simulink model "ClosedLoop_ACCsim"  (Simulink 9.2)
settings: Solver=VariableStepAuto  StartTime=0.0  StopTime=5  RelTol=1e-3
libraries: neural x533
(part 10 of 24)

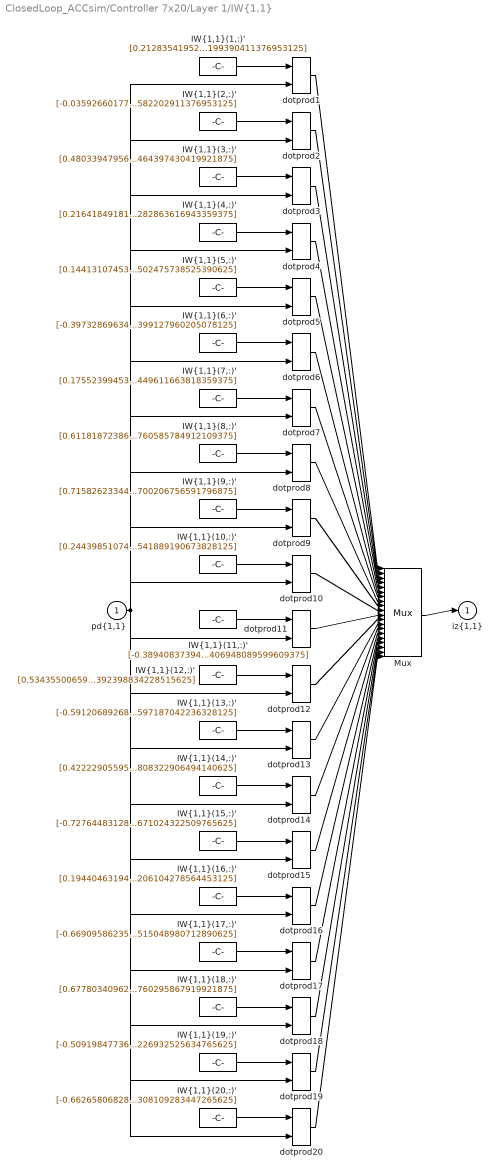
== system ClosedLoop_ACCsim/Controller 7x20/Layer 1/IW{1,1} ==
  "pd{1,1}" : Inport  PortDimensions=5
      mask Display: e = 0.06;c1 = [120 230 180]/255;c2 = ([120 230 180]+0)/(256+128);c3 = ([120 230 180]+128)/(256+128);patch([0 1 1 0],[0 0 1 1],c1);patch([0 1 1 1-e 1-e 0+e],[0 0 1 1-e 0+e 0+e],c2);patch([0 0 1 1-e 0+e 0+e],[0 1 1 1-e 1-e 0+e],c3);plot([0 1 1 0 0],[0 0 1 1 0]);
  "IW{1,1}(1,:)'" : Constant  Value=[0.212835419521011315335812241755775175988674163818359375;-0.3927359580132747662872816363233141601085662841796875;-0.144152301067769827991327247218578122556209564208984375;-0.58889119361664221674601549239014275372028350830078125;-0.034369251210462976875437135504398611374199390411376953125]
      mask Display: e = 0.06;c1 = [120 150 230]/255;c2 = ([120 150 230]+0)/383;c3 = ([120 150 230]+128)/383;patch([0 1 1 0],[0 0 1 1],c1);patch([0 1 1 1-e 1-e 0+e],[0 0 1 1-e 0+e 0+e],c2);patch([0 0 1 1-e 0+e 0+e],[0 1 1 1-e 1-e 0+e],c3);plot([0 1 1 0 0],[0 0 1 1 0]);disp('Weights');
  "IW{1,1}(10,:)'" : Constant  Value=[0.2443985107421249580728073169666458852589130401611328125;0.251248156472832884222867733114981092512607574462890625;0.12802800348474974168055950940470211207866668701171875;0.5142082099368210368339759952505119144916534423828125;0.295116604969453633078302345893462188541889190673828125]
      mask Display: e = 0.06;c1 = [120 150 230]/255;c2 = ([120 150 230]+0)/383;c3 = ([120 150 230]+128)/383;patch([0 1 1 0],[0 0 1 1],c1);patch([0 1 1 1-e 1-e 0+e],[0 0 1 1-e 0+e 0+e],c2);patch([0 0 1 1-e 0+e 0+e],[0 1 1 1-e 1-e 0+e],c3);plot([0 1 1 0 0],[0 0 1 1 0]);disp('Weights');
  "IW{1,1}(11,:)'" : Constant  Value=[-0.389408373941988517064061170458444394171237945556640625;-0.5598485732379170354278130616876296699047088623046875;0.18512337722791460947746600140817463397979736328125;0.15592881193242147386257556718192063271999359130859375;-0.56991107693016029855925808078609406948089599609375]
      mask Display: e = 0.06;c1 = [120 150 230]/255;c2 = ([120 150 230]+0)/383;c3 = ([120 150 230]+128)/383;patch([0 1 1 0],[0 0 1 1],c1);patch([0 1 1 1-e 1-e 0+e],[0 0 1 1-e 0+e 0+e],c2);patch([0 0 1 1-e 0+e 0+e],[0 1 1 1-e 1-e 0+e],c3);plot([0 1 1 0 0],[0 0 1 1 0]);disp('Weights');
  "IW{1,1}(12,:)'" : Constant  Value=[0.5343550065999895792856477783061563968658447265625;0.250744758001088363652542057025129906833171844482421875;-0.461235807435400213538656544187688268721103668212890625;0.1640473631794022446594993880353285931050777435302734375;0.67067318966512046163330751369358040392398834228515625]
      mask Display: e = 0.06;c1 = [120 150 230]/255;c2 = ([120 150 230]+0)/383;c3 = ([120 150 230]+128)/383;patch([0 1 1 0],[0 0 1 1],c1);patch([0 1 1 1-e 1-e 0+e],[0 0 1 1-e 0+e 0+e],c2);patch([0 0 1 1-e 0+e 0+e],[0 1 1 1-e 1-e 0+e],c3);plot([0 1 1 0 0],[0 0 1 1 0]);disp('Weights');
  "IW{1,1}(13,:)'" : Constant  Value=[-0.5912068926854825434702433994971215724945068359375;-0.2038470656672795866537484243963262997567653656005859375;-0.1583124425194095408198080576767097227275371551513671875;-0.486613579148853225841975245202775113284587860107421875;-0.1335803269614399824138928352112998254597187042236328125]
      mask Display: e = 0.06;c1 = [120 150 230]/255;c2 = ([120 150 230]+0)/383;c3 = ([120 150 230]+128)/383;patch([0 1 1 0],[0 0 1 1],c1);patch([0 1 1 1-e 1-e 0+e],[0 0 1 1-e 0+e 0+e],c2);patch([0 0 1 1-e 0+e 0+e],[0 1 1 1-e 1-e 0+e],c3);plot([0 1 1 0 0],[0 0 1 1 0]);disp('Weights');
  "IW{1,1}(14,:)'" : Constant  Value=[0.4222290559586252545187790019554086029529571533203125;0.589193425221622657517173138330690562725067138671875;0.5154792487456205662965658120810985565185546875;-0.44820131779535354876742303531500510871410369873046875;-0.028408822728697803727815340835149982012808322906494140625]
      mask Display: e = 0.06;c1 = [120 150 230]/255;c2 = ([120 150 230]+0)/383;c3 = ([120 150 230]+128)/383;patch([0 1 1 0],[0 0 1 1],c1);patch([0 1 1 1-e 1-e 0+e],[0 0 1 1-e 0+e 0+e],c2);patch([0 0 1 1-e 0+e 0+e],[0 1 1 1-e 1-e 0+e],c3);plot([0 1 1 0 0],[0 0 1 1 0]);disp('Weights');
  "IW{1,1}(15,:)'" : Constant  Value=[-0.72764483128828494340467614165390841662883758544921875;0.76631521718359596473391093240934424102306365966796875;-0.261586670059799575316361597288050688803195953369140625;0.26312492002977949656639111708500422537326812744140625;0.90935896357760359620669987634755671024322509765625]
      mask Display: e = 0.06;c1 = [120 150 230]/255;c2 = ([120 150 230]+0)/383;c3 = ([120 150 230]+128)/383;patch([0 1 1 0],[0 0 1 1],c1);patch([0 1 1 1-e 1-e 0+e],[0 0 1 1-e 0+e 0+e],c2);patch([0 0 1 1-e 0+e 0+e],[0 1 1 1-e 1-e 0+e],c3);plot([0 1 1 0 0],[0 0 1 1 0]);disp('Weights');
  "IW{1,1}(16,:)'" : Constant  Value=[0.194404631947168893280064594364375807344913482666015625;0.5552546495174126572891282194177620112895965576171875;0.058508554392630300611255478315797518007457256317138671875;-0.27216863837114579904863376214052550494670867919921875;0.7418254711021508018831127628800459206104278564453125]
      mask Display: e = 0.06;c1 = [120 150 230]/255;c2 = ([120 150 230]+0)/383;c3 = ([120 150 230]+128)/383;patch([0 1 1 0],[0 0 1 1],c1);patch([0 1 1 1-e 1-e 0+e],[0 0 1 1-e 0+e 0+e],c2);patch([0 0 1 1-e 0+e 0+e],[0 1 1 1-e 1-e 0+e],c3);plot([0 1 1 0 0],[0 0 1 1 0]);disp('Weights');
  "IW{1,1}(17,:)'" : Constant  Value=[-0.6690958623540581573507779467036016285419464111328125;0.414850507163107007357893962762318551540374755859375;0.36526786443267000858980964039801619946956634521484375;0.066989067247426092865936197995324619114398956298828125;0.492191258252048735588601857671164907515048980712890625]
      mask Display: e = 0.06;c1 = [120 150 230]/255;c2 = ([120 150 230]+0)/383;c3 = ([120 150 230]+128)/383;patch([0 1 1 0],[0 0 1 1],c1);patch([0 1 1 1-e 1-e 0+e],[0 0 1 1-e 0+e 0+e],c2);patch([0 0 1 1-e 0+e 0+e],[0 1 1 1-e 1-e 0+e],c3);plot([0 1 1 0 0],[0 0 1 1 0]);disp('Weights');
  "IW{1,1}(18,:)'" : Constant  Value=[0.67780340962930984982648396908189170062541961669921875;-0.166200801785160667822793811865267343819141387939453125;0.007773451654268163750483022766957219573669135570526123046875;-0.6277118496053983864868541786563582718372344970703125;-0.10179050764502566017721818525387789122760295867919921875]
      mask Display: e = 0.06;c1 = [120 150 230]/255;c2 = ([120 150 230]+0)/383;c3 = ([120 150 230]+128)/383;patch([0 1 1 0],[0 0 1 1],c1);patch([0 1 1 1-e 1-e 0+e],[0 0 1 1-e 0+e 0+e],c2);patch([0 0 1 1-e 0+e 0+e],[0 1 1 1-e 1-e 0+e],c3);plot([0 1 1 0 0],[0 0 1 1 0]);disp('Weights');
  "IW{1,1}(19,:)'" : Constant  Value=[-0.50919847736597778631306709939963184297084808349609375;0.29458849558637767440671950680552981793880462646484375;0.6164242054481239296848116282490082085132598876953125;-0.05022444481905320723402752491892897523939609527587890625;0.56929857309828568734388909433619119226932525634765625]
      mask Display: e = 0.06;c1 = [120 150 230]/255;c2 = ([120 150 230]+0)/383;c3 = ([120 150 230]+128)/383;patch([0 1 1 0],[0 0 1 1],c1);patch([0 1 1 1-e 1-e 0+e],[0 0 1 1-e 0+e 0+e],c2);patch([0 0 1 1-e 0+e 0+e],[0 1 1 1-e 1-e 0+e],c3);plot([0 1 1 0 0],[0 0 1 1 0]);disp('Weights');
  "IW{1,1}(2,:)'" : Constant  Value=[-0.035926601776865262072302442675209022127091884613037109375;0.341274893573676296743002467337646521627902984619140625;-0.1624957466411529605210262161563150584697723388671875;0.68546422590090638760074170932057313621044158935546875;-0.76852906292452705105944232855108566582202911376953125]
      mask Display: e = 0.06;c1 = [120 150 230]/255;c2 = ([120 150 230]+0)/383;c3 = ([120 150 230]+128)/383;patch([0 1 1 0],[0 0 1 1],c1);patch([0 1 1 1-e 1-e 0+e],[0 0 1 1-e 0+e 0+e],c2);patch([0 0 1 1-e 0+e 0+e],[0 1 1 1-e 1-e 0+e],c3);plot([0 1 1 0 0],[0 0 1 1 0]);disp('Weights');
  "IW{1,1}(20,:)'" : Constant  Value=[-0.66265806828597562105898077788879163563251495361328125;-0.8358574702130796563182002500980161130428314208984375;0.332826348998758014818832862147246487438678741455078125;0.75074131206823901951707966873073019087314605712890625;-0.1851004659156537945907672337853000499308109283447265625]
      mask Display: e = 0.06;c1 = [120 150 230]/255;c2 = ([120 150 230]+0)/383;c3 = ([120 150 230]+128)/383;patch([0 1 1 0],[0 0 1 1],c1);patch([0 1 1 1-e 1-e 0+e],[0 0 1 1-e 0+e 0+e],c2);patch([0 0 1 1-e 0+e 0+e],[0 1 1 1-e 1-e 0+e],c3);plot([0 1 1 0 0],[0 0 1 1 0]);disp('Weights');
  "IW{1,1}(3,:)'" : Constant  Value=[0.480339479563791471594669246769626624882221221923828125;-0.59592850278037456934754345638793893158435821533203125;-0.1930903352979157772129070735900313593447208404541015625;0.114496074419272619859810902198660187423229217529296875;-0.361143691370916009031333260281826369464397430419921875]
      mask Display: e = 0.06;c1 = [120 150 230]/255;c2 = ([120 150 230]+0)/383;c3 = ([120 150 230]+128)/383;patch([0 1 1 0],[0 0 1 1],c1);patch([0 1 1 1-e 1-e 0+e],[0 0 1 1-e 0+e 0+e],c2);patch([0 0 1 1-e 0+e 0+e],[0 1 1 1-e 1-e 0+e],c3);plot([0 1 1 0 0],[0 0 1 1 0]);disp('Weights');
  "IW{1,1}(4,:)'" : Constant  Value=[0.2164184918114815114886795299753430299460887908935546875;0.9400873566467999875584382607485167682170867919921875;-0.303205328969188225851638662788900546729564666748046875;-0.44570874540381921757870031797210685908794403076171875;0.18120949337870850825993329635821282863616943359375]
      mask Display: e = 0.06;c1 = [120 150 230]/255;c2 = ([120 150 230]+0)/383;c3 = ([120 150 230]+128)/383;patch([0 1 1 0],[0 0 1 1],c1);patch([0 1 1 1-e 1-e 0+e],[0 0 1 1-e 0+e 0+e],c2);patch([0 0 1 1-e 0+e 0+e],[0 1 1 1-e 1-e 0+e],c3);plot([0 1 1 0 0],[0 0 1 1 0]);disp('Weights');
  "IW{1,1}(5,:)'" : Constant  Value=[0.1441310745332750331559878986809053458273410797119140625;-0.9206317506257928329205242334865033626556396484375;-0.4099304221757520405589048095862381160259246826171875;-0.568009386779689151580896577797830104827880859375;0.344113066470443096367404223201447166502475738525390625]
      mask Display: e = 0.06;c1 = [120 150 230]/255;c2 = ([120 150 230]+0)/383;c3 = ([120 150 230]+128)/383;patch([0 1 1 0],[0 0 1 1],c1);patch([0 1 1 1-e 1-e 0+e],[0 0 1 1-e 0+e 0+e],c2);patch([0 0 1 1-e 0+e 0+e],[0 1 1 1-e 1-e 0+e],c3);plot([0 1 1 0 0],[0 0 1 1 0]);disp('Weights');
  "IW{1,1}(6,:)'" : Constant  Value=[-0.397328696346857801469099058522260747849941253662109375;-0.0029566435601016071398061679786906097433529794216156005859375;0.4309051632885638749570489380857907235622406005859375;-0.67053491722794689167130854912102222442626953125;-0.466971235009332463761211329256184399127960205078125]
      mask Display: e = 0.06;c1 = [120 150 230]/255;c2 = ([120 150 230]+0)/383;c3 = ([120 150 230]+128)/383;patch([0 1 1 0],[0 0 1 1],c1);patch([0 1 1 1-e 1-e 0+e],[0 0 1 1-e 0+e 0+e],c2);patch([0 0 1 1-e 0+e 0+e],[0 1 1 1-e 1-e 0+e],c3);plot([0 1 1 0 0],[0 0 1 1 0]);disp('Weights');
  "IW{1,1}(7,:)'" : Constant  Value=[0.175523994536887883999298765047569759190082550048828125;0.2783338599097124888004373133298940956592559814453125;0.67569683197213648018220055746496655046939849853515625;-0.84534829514369536074269717573770321905612945556640625;0.08340677879841050523790357829057029448449611663818359375]
      mask Display: e = 0.06;c1 = [120 150 230]/255;c2 = ([120 150 230]+0)/383;c3 = ([120 150 230]+128)/383;patch([0 1 1 0],[0 0 1 1],c1);patch([0 1 1 1-e 1-e 0+e],[0 0 1 1-e 0+e 0+e],c2);patch([0 0 1 1-e 0+e 0+e],[0 1 1 1-e 1-e 0+e],c3);plot([0 1 1 0 0],[0 0 1 1 0]);disp('Weights');
  "IW{1,1}(8,:)'" : Constant  Value=[0.61181872386841373856469772363197989761829376220703125;-0.201160270514594896607007967759273014962673187255859375;0.377397473828878116108853646437637507915496826171875;-0.22875332743301834970139907454722560942173004150390625;0.1859440325483736611289486972964368760585784912109375]
      mask Display: e = 0.06;c1 = [120 150 230]/255;c2 = ([120 150 230]+0)/383;c3 = ([120 150 230]+128)/383;patch([0 1 1 0],[0 0 1 1],c1);patch([0 1 1 1-e 1-e 0+e],[0 0 1 1-e 0+e 0+e],c2);patch([0 0 1 1-e 0+e 0+e],[0 1 1 1-e 1-e 0+e],c3);plot([0 1 1 0 0],[0 0 1 1 0]);disp('Weights');
  "IW{1,1}(9,:)'" : Constant  Value=[0.71582623344398610409911043461761437356472015380859375;-0.897528066616040565151024566148407757282257080078125;-0.715669583388752972297197629814036190509796142578125;0.052208333596294072276311482028177124448120594024658203125;0.254905335750240158443347127104061655700206756591796875]
      mask Display: e = 0.06;c1 = [120 150 230]/255;c2 = ([120 150 230]+0)/383;c3 = ([120 150 230]+128)/383;patch([0 1 1 0],[0 0 1 1],c1);patch([0 1 1 1-e 1-e 0+e],[0 0 1 1-e 0+e 0+e],c2);patch([0 0 1 1-e 0+e 0+e],[0 1 1 1-e 1-e 0+e],c3);plot([0 1 1 0 0],[0 0 1 1 0]);disp('Weights');
  Mux : Mux  Inputs=20
      mask Display: e = 0.06;c1 = [120 150 230]/255;c2 = ([120 150 230]+0)/383;c3 = ([120 150 230]+128)/383;patch([0 1 1 0],[0 0 1 1],c1);patch([0 1 1 1-e 1-e 0+e],[0 0 1 1-e 0+e 0+e],c2);patch([0 0 1 1-e 0+e 0+e],[0 1 1 1-e 1-e 0+e],c3);plot([0 1 1 0 0],[0 0 1 1 0]);disp('Mux');
  dotprod{1..20} (20 alike) : neural/Weight Functions/dotprod
  "iz{1,1}" : Outport
      mask Display: e = 0.06;c1 = [120 230 180]/255;c2 = ([120 230 180]+0)/(256+128);c3 = ([120 230 180]+128)/(256+128);patch([0 1 1 0],[0 0 1 1],c1);patch([0 1 1 1-e 1-e 0+e],[0 0 1 1-e 0+e 0+e],c2);patch([0 0 1 1-e 0+e 0+e],[0 1 1 1-e 1-e 0+e],c3);plot([0 1 1 0 0],[0 0 1 1 0]);
  wires:
  Mux/1 -> "iz{1,1}"/1
  dotprod20/1 -> Mux/20
  "IW{1,1}(20,:)'"/1 -> dotprod20/1
  dotprod19/1 -> Mux/19
  "IW{1,1}(19,:)'"/1 -> dotprod19/1
  dotprod18/1 -> Mux/18
  "IW{1,1}(18,:)'"/1 -> dotprod18/1
  dotprod17/1 -> Mux/17
  "IW{1,1}(17,:)'"/1 -> dotprod17/1
  dotprod16/1 -> Mux/16
  "IW{1,1}(16,:)'"/1 -> dotprod16/1
  dotprod15/1 -> Mux/15
  "IW{1,1}(15,:)'"/1 -> dotprod15/1
  dotprod14/1 -> Mux/14
  "IW{1,1}(14,:)'"/1 -> dotprod14/1
  dotprod13/1 -> Mux/13
  "IW{1,1}(13,:)'"/1 -> dotprod13/1
  dotprod12/1 -> Mux/12
  "IW{1,1}(12,:)'"/1 -> dotprod12/1
  dotprod11/1 -> Mux/11
  "IW{1,1}(11,:)'"/1 -> dotprod11/1
  dotprod10/1 -> Mux/10
  "IW{1,1}(10,:)'"/1 -> dotprod10/1
  dotprod9/1 -> Mux/9
  "IW{1,1}(9,:)'"/1 -> dotprod9/1
  dotprod8/1 -> Mux/8
  "IW{1,1}(8,:)'"/1 -> dotprod8/1
  dotprod7/1 -> Mux/7
  "IW{1,1}(7,:)'"/1 -> dotprod7/1
  dotprod6/1 -> Mux/6
  "IW{1,1}(6,:)'"/1 -> dotprod6/1
  dotprod5/1 -> Mux/5
  "IW{1,1}(5,:)'"/1 -> dotprod5/1
  dotprod4/1 -> Mux/4
  "IW{1,1}(4,:)'"/1 -> dotprod4/1
  dotprod3/1 -> Mux/3
  "IW{1,1}(3,:)'"/1 -> dotprod3/1
  dotprod2/1 -> Mux/2
  "IW{1,1}(2,:)'"/1 -> dotprod2/1
  dotprod1/1 -> Mux/1
  "pd{1,1}"/1 -> dotprod20/2, dotprod19/2, dotprod18/2, dotprod17/2, dotprod16/2, dotprod15/2, dotprod14/2, dotprod13/2, dotprod12/2, dotprod11/2, dotprod10/2, dotprod9/2, dotprod8/2, dotprod7/2, dotprod6/2, dotprod5/2, dotprod4/2, dotprod3/2, dotprod2/2, dotprod1/2
  "IW{1,1}(1,:)'"/1 -> dotprod1/1

== system ClosedLoop_ACCsim/Controller 7x20/Layer 2/Delays 1 ==
  "p{2}" : Inport  PortDimensions=20
      mask Display: e = 0.06;c1 = [120 230 180]/255;c2 = ([120 230 180]+0)/(256+128);c3 = ([120 230 180]+128)/(256+128);patch([0 1 1 0],[0 0 1 1],c1);patch([0 1 1 1-e 1-e 0+e],[0 0 1 1-e 0+e 0+e],c2);patch([0 0 1 1-e 0+e 0+e],[0 1 1 1-e 1-e 0+e],c3);plot([0 1 1 0 0],[0 0 1 1 0]);
  mux : Mux  Inputs=1
      mask Display: e = 0.06;c1 = [120 150 230]/255;c2 = ([120 150 230]+0)/383;c3 = ([120 150 230]+128)/383;patch([0 1 1 0],[0 0 1 1],c1);patch([0 1 1 1-e 1-e 0+e],[0 0 1 1-e 0+e 0+e],c2);patch([0 0 1 1-e 0+e 0+e],[0 1 1 1-e 1-e 0+e],c3);plot([0 1 1 0 0],[0 0 1 1 0]);disp('Mux')
  "pd{2,1}" : Outport
      mask Display: e = 0.06;c1 = [120 230 180]/255;c2 = ([120 230 180]+0)/(256+128);c3 = ([120 230 180]+128)/(256+128);patch([0 1 1 0],[0 0 1 1],c1);patch([0 1 1 1-e 1-e 0+e],[0 0 1 1-e 0+e 0+e],c2);patch([0 0 1 1-e 0+e 0+e],[0 1 1 1-e 1-e 0+e],c3);plot([0 1 1 0 0],[0 0 1 1 0]);
  wires:
  mux/1 -> "pd{2,1}"/1
  "p{2}"/1 -> mux/1

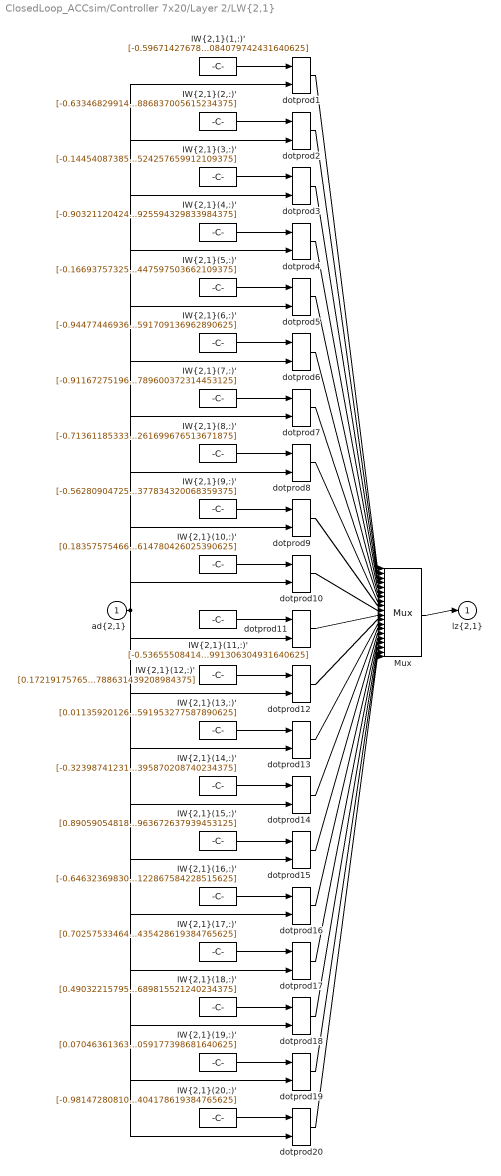
== system ClosedLoop_ACCsim/Controller 7x20/Layer 2/LW{2,1} ==
  "ad{2,1}" : Inport  PortDimensions=20
      mask Display: e = 0.06;c1 = [120 230 180]/255;c2 = ([120 230 180]+0)/(256+128);c3 = ([120 230 180]+128)/(256+128);patch([0 1 1 0],[0 0 1 1],c1);patch([0 1 1 1-e 1-e 0+e],[0 0 1 1-e 0+e 0+e],c2);patch([0 0 1 1-e 0+e 0+e],[0 1 1 1-e 1-e 0+e],c3);plot([0 1 1 0 0],[0 0 1 1 0]);
  "IW{2,1}(1,:)'" : Constant  Value=[-0.596714276780772490127446872065775096416473388671875;-0.4730965696108437867906104656867682933807373046875;-0.3754862846921918073661572634591720998287200927734375;0.826107146757460331087941085570491850376129150390625;0.68765324578509734454456747698714025318622589111328125;-0.2482387120107035494154246180187328718602657318115234375;-0.6288666858010956151048276296933181583881378173828125;-0.227092772737665538063112080635619349777698516845703125;-0.448416230017323280687691067214473150670528411865234375;-0.3102895805729553035945400552009232342243194580078125;0.8686495588796068201276057152426801621913909912109375;-0.5228732621141178871226884439238347113132476806640625;0.381787072232372015623269589923438616096973419189453125;0.937937844531308684281611931510269641876220703125;0.663677390184762572289400850422680377960205078125;-0.399666395705869537113841261088964529335498809814453125;-0.9388917382288408663981726931524462997913360595703125;-0.145080590252849417343128379798145033419132232666015625;-0.23328604154895848932227409022743813693523406982421875;-0.4950018876128583489304446629830636084079742431640625]
      mask Display: e = 0.06;c1 = [120 150 230]/255;c2 = ([120 150 230]+0)/383;c3 = ([120 150 230]+128)/383;patch([0 1 1 0],[0 0 1 1],c1);patch([0 1 1 1-e 1-e 0+e],[0 0 1 1-e 0+e 0+e],c2);patch([0 0 1 1-e 0+e 0+e],[0 1 1 1-e 1-e 0+e],c3);plot([0 1 1 0 0],[0 0 1 1 0]);disp('weights');
  "IW{2,1}(10,:)'" : Constant  Value=[0.183575754664555390593960737533052451908588409423828125;-0.847982673417647436764355006744153797626495361328125;-0.74751903679590814277844401658512651920318603515625;-0.2370716772188005416754918996957712806761264801025390625;-0.133567434904125204031544171812129206955432891845703125;-0.259892873902302257160812359870760701596736907958984375;-0.055934491627692033144381156262170406989753246307373046875;-0.27070482054377886793616880822810344398021697998046875;0.53296842534778132716155596426688134670257568359375;-0.7362598073046588975643089725053869187831878662109375;-0.04283030361047768241888888951507396996021270751953125;0.6447845216517695821067945871618576347827911376953125;-0.324343651727461879108460607312736101448535919189453125;-0.75886261287393785845978300130809657275676727294921875;0.71490590352001837093354197349981404840946197509765625;0.29995835854936159226014069645316340029239654541015625;0.95404815169850365474957243350218050181865692138671875;0.71447560503657914221520286446320824325084686279296875;-0.1812139934022258536128191508396412245929241180419921875;0.29314938996913841862124172621406614780426025390625]
      mask Display: e = 0.06;c1 = [120 150 230]/255;c2 = ([120 150 230]+0)/383;c3 = ([120 150 230]+128)/383;patch([0 1 1 0],[0 0 1 1],c1);patch([0 1 1 1-e 1-e 0+e],[0 0 1 1-e 0+e 0+e],c2);patch([0 0 1 1-e 0+e 0+e],[0 1 1 1-e 1-e 0+e],c3);plot([0 1 1 0 0],[0 0 1 1 0]);disp('weights');
  "IW{2,1}(11,:)'" : Constant  Value=[-0.536555084148062189086658690939657390117645263671875;0.1742134412923512787330082574044354259967803955078125;-0.1091841483734883322398445670842193067073822021484375;-0.127758394510482542472118439036421477794647216796875;0.0710052871003028496232900579343549907207489013671875;-0.4233643555650024037362300077802501618862152099609375;-0.990372379820247061843474511988461017608642578125;-0.8053736847920609509543510284856893122196197509765625;-0.0524893401012906934965940308757126331329345703125;-0.7182283047005337817125791843864135444164276123046875;0.4516862057392743157180348134716041386127471923828125;0.2512959871288391600074874077108688652515411376953125;0.9975125668869291306606328362249769270420074462890625;0.017789158581016817350928249652497470378875732421875;0.694734021325817518999201638507656753063201904296875;-0.4027442532772458338996557358768768608570098876953125;-0.6693679102871621378056943285628221929073333740234375;-0.848006570175071860973048387677408754825592041015625;-0.9171870242482729196353830047883093357086181640625;-0.9294145428148059551176629611290991306304931640625]
      mask Display: e = 0.06;c1 = [120 150 230]/255;c2 = ([120 150 230]+0)/383;c3 = ([120 150 230]+128)/383;patch([0 1 1 0],[0 0 1 1],c1);patch([0 1 1 1-e 1-e 0+e],[0 0 1 1-e 0+e 0+e],c2);patch([0 0 1 1-e 0+e 0+e],[0 1 1 1-e 1-e 0+e],c3);plot([0 1 1 0 0],[0 0 1 1 0]);disp('weights');
  "IW{2,1}(12,:)'" : Constant  Value=[0.172191757651370902504339710503700189292430877685546875;0.2640539786435167624034647815278731286525726318359375;-0.1351094653078728224926408074679784476757049560546875;0.265679924954510815471309115309850312769412994384765625;0.6238274556803877768373922663158737123012542724609375;-0.5798310442620191462737011534045450389385223388671875;-0.1796278474227658017436937143429531715810298919677734375;0.71619231256662752027608576099737547338008880615234375;0.65624553128959883796511576292687095701694488525390625;-0.8849024976104440387558724978589452803134918212890625;-0.800773851320517593421755009330809116363525390625;-0.600915230860560978243256613495759665966033935546875;-0.372946487868269394017062268176232464611530303955078125;-0.76185671720366354708886547086876817047595977783203125;-0.446289087096395975517992837922065518796443939208984375;0.8955737820295512907620150144794024527072906494140625;0.588088386367795035170047412975691258907318115234375;-0.90249064211068574792307117604650557041168212890625;0.201458342102948051444144539345870725810527801513671875;0.5969729216284009876147820250480435788631439208984375]
      mask Display: e = 0.06;c1 = [120 150 230]/255;c2 = ([120 150 230]+0)/383;c3 = ([120 150 230]+128)/383;patch([0 1 1 0],[0 0 1 1],c1);patch([0 1 1 1-e 1-e 0+e],[0 0 1 1-e 0+e 0+e],c2);patch([0 0 1 1-e 0+e 0+e],[0 1 1 1-e 1-e 0+e],c3);plot([0 1 1 0 0],[0 0 1 1 0]);disp('weights');
  "IW{2,1}(13,:)'" : Constant  Value=[0.01135920126168527867493995842096410342492163181304931640625;-0.6752045122749044114840444308356381952762603759765625;0.47809423110813964452603386234841309487819671630859375;-0.725206068689159710771718891919590532779693603515625;0.95242291194894035388784914175630547106266021728515625;0.835481818378403406910592821077443659305572509765625;0.825970710134531049817496750620193779468536376953125;-0.4109093858092716100571806236985139548778533935546875;0.79293378494690147650914013865985907614231109619140625;0.1959338686218536629279896033040131442248821258544921875;-0.08866817270302672360227091985507286153733730316162109375;-0.96052455900604150063060160391614772379398345947265625;0.75780958880128623800231935092597268521785736083984375;-0.188713694066320047948437377272057346999645233154296875;-0.1935733069548523921366012245925958268344402313232421875;0.5368728690040824869100788419018499553203582763671875;-0.33624025202435936510170222391025163233280181884765625;-0.2054555943188327293835726550241815857589244842529296875;0.40632669121950260038289570729830302298069000244140625;-1.0112486178900932376478749574744142591953277587890625]
      mask Display: e = 0.06;c1 = [120 150 230]/255;c2 = ([120 150 230]+0)/383;c3 = ([120 150 230]+128)/383;patch([0 1 1 0],[0 0 1 1],c1);patch([0 1 1 1-e 1-e 0+e],[0 0 1 1-e 0+e 0+e],c2);patch([0 0 1 1-e 0+e 0+e],[0 1 1 1-e 1-e 0+e],c3);plot([0 1 1 0 0],[0 0 1 1 0]);disp('weights');
  "IW{2,1}(14,:)'" : Constant  Value=[-0.3239874123125667804146132766618393361568450927734375;0.4881418309743406069856064277701079845428466796875;0.326669464605274739721352261767606250941753387451171875;0.1307749349082021061985159349205787293612957000732421875;-0.235189082410515393206651424407027661800384521484375;-0.173503183993380993843658188779954798519611358642578125;-0.62307338183625116112551722835632972419261932373046875;0.359619714582356364562798489714623428881168365478515625;-0.86543219516158609305733762084855698049068450927734375;0.157672390941171303158085947870858944952487945556640625;-0.0737133145161684433244175806976272724568843841552734375;-0.60377629083127948295128817335353232920169830322265625;0.395332681982889511118628433905541896820068359375;-0.1940607512643813536978854017434059642255306243896484375;0.748436546441429317866322890040464699268341064453125;0.6740533075742429769405816841754131019115447998046875;0.02712699063560593260024944584074546582996845245361328125;-0.699355682720601112833946899627335369586944580078125;0.582122220716618787861307282582856714725494384765625;-0.37172402538469506705354206133051775395870208740234375]
      mask Display: e = 0.06;c1 = [120 150 230]/255;c2 = ([120 150 230]+0)/383;c3 = ([120 150 230]+128)/383;patch([0 1 1 0],[0 0 1 1],c1);patch([0 1 1 1-e 1-e 0+e],[0 0 1 1-e 0+e 0+e],c2);patch([0 0 1 1-e 0+e 0+e],[0 1 1 1-e 1-e 0+e],c3);plot([0 1 1 0 0],[0 0 1 1 0]);disp('weights');
  "IW{2,1}(15,:)'" : Constant  Value=[0.8905905481823761515869364302488975226879119873046875;0.060763325283351134198372989203562610782682895660400390625;0.01395975094303837822640179666677795466966927051544189453125;-0.406676748190684833605956782776047475636005401611328125;-0.54024093716630883221796466386877000331878662109375;-0.6139953812401193200543048078543506562709808349609375;0.598163458314731055764923439710400998592376708984375;-0.267005194052315764086102944929734803736209869384765625;0.469349291878817354017883189953863620758056640625;-0.1296558887726406428253511649018037132918834686279296875;0.639120470181471223014568749931640923023223876953125;-0.340341201703816154111592595654656179249286651611328125;-0.78436319489527173143272875677212141454219818115234375;-0.28079682508502823434781703326734714210033416748046875;0.66665878258287281088456666111596859991550445556640625;0.391027589242355866350209225856815464794635772705078125;-0.58865835049580750304443199638626538217067718505859375;0.44174127439099730718652381256106309592723846435546875;-0.64491616669480522627821983405738137662410736083984375;0.04178499131185919868158862300333566963672637939453125]
      mask Display: e = 0.06;c1 = [120 150 230]/255;c2 = ([120 150 230]+0)/383;c3 = ([120 150 230]+128)/383;patch([0 1 1 0],[0 0 1 1],c1);patch([0 1 1 1-e 1-e 0+e],[0 0 1 1-e 0+e 0+e],c2);patch([0 0 1 1-e 0+e 0+e],[0 1 1 1-e 1-e 0+e],c3);plot([0 1 1 0 0],[0 0 1 1 0]);disp('weights');
  "IW{2,1}(16,:)'" : Constant  Value=[-0.64632369830492242268604741184390150010585784912109375;-0.47702812309863384943042774466448463499546051025390625;-0.621982623401258205575459214742295444011688232421875;-0.8986889077679769410877952395821921527385711669921875;0.93691434754725400058106288270209915935993194580078125;0.098627638124162697597085980305564589798450469970703125;-0.3394235065495985192995931356563232839107513427734375;0.29237217744259391682959403624408878386020660400390625;-0.063848896990207293367092233893345110118389129638671875;-0.91817548776264501508848070443491451442241668701171875;0.75494077117864488712939419201575219631195068359375;0.497085785391184920012364045760477893054485321044921875;-0.026150924336305413075987047477610758505761623382568359375;0.9411932795034083643059830137644894421100616455078125;-0.90053191767845797155445097814663313329219818115234375;0.66303578335757951123241582536138594150543212890625;-0.83065193999175945815949262396316044032573699951171875;-0.9890885557359532231913590294425375759601593017578125;0.3357477342207342285718141283723525702953338623046875;-0.88466201619057172056415083716274239122867584228515625]
      mask Display: e = 0.06;c1 = [120 150 230]/255;c2 = ([120 150 230]+0)/383;c3 = ([120 150 230]+128)/383;patch([0 1 1 0],[0 0 1 1],c1);patch([0 1 1 1-e 1-e 0+e],[0 0 1 1-e 0+e 0+e],c2);patch([0 0 1 1-e 0+e 0+e],[0 1 1 1-e 1-e 0+e],c3);plot([0 1 1 0 0],[0 0 1 1 0]);disp('weights');
  "IW{2,1}(17,:)'" : Constant  Value=[0.7025753346407059840572628672816790640354156494140625;-0.3770567280982621838347768061794340610504150390625;-0.6860655094816063837015462922863662242889404296875;-0.72803056045027059184349127463065087795257568359375;0.3598736062536123103683394219842739403247833251953125;-0.9389672098291452773111132046324200928211212158203125;-0.43684369829937441664924335782416164875030517578125;-0.4780002083518282152141409824253059923648834228515625;0.1823875310058855614414596857386641204357147216796875;-0.681497637395278577088220117730088531970977783203125;-0.2973393965556956342055627828813157975673675537109375;0.54596063508257142160573494038544595241546630859375;0.3538108683173948332267855221289210021495819091796875;0.7389844587913112494703682386898435652256011962890625;-0.556587704700358898435297305695712566375732421875;-0.18968495961943165895036145229823887348175048828125;0.72344062941002817979097017087042331695556640625;-0.8075569237866730976094231664319522678852081298828125;-0.3858498423559526546711140326806344091892242431640625;-0.130481398489755040515092332498170435428619384765625]
      mask Display: e = 0.06;c1 = [120 150 230]/255;c2 = ([120 150 230]+0)/383;c3 = ([120 150 230]+128)/383;patch([0 1 1 0],[0 0 1 1],c1);patch([0 1 1 1-e 1-e 0+e],[0 0 1 1-e 0+e 0+e],c2);patch([0 0 1 1-e 0+e 0+e],[0 1 1 1-e 1-e 0+e],c3);plot([0 1 1 0 0],[0 0 1 1 0]);disp('weights');
  "IW{2,1}(18,:)'" : Constant  Value=[0.490322157956438242631946877736481837928295135498046875;0.4758346644900777189235441255732439458370208740234375;-0.121823626398499140766062964758020825684070587158203125;-0.283238333464887415136246318070334382355213165283203125;0.87995601661929701009512427845038473606109619140625;-0.0131294477643324990212558844859813689254224300384521484375;-0.1145305937346700886347861114700208418071269989013671875;-0.36898502082857909112334482415462844073772430419921875;0.87855306445759839828468784617143683135509490966796875;0.01504193846796410445609826211921244976110756397247314453125;-0.3759568394249319656097441111342050135135650634765625;-0.83115694525920613688896310122800059616565704345703125;-0.1886683992374456331209131576542858965694904327392578125;0.96530058523640371870300214141025207936763763427734375;-0.81454786747062224439019928468042053282260894775390625;-0.81790376939442321901907462233793921768665313720703125;-0.81443554761264869146231148988590575754642486572265625;-0.06667660935967055502171518810428096912801265716552734375;-0.153202194490143328575726400231360457837581634521484375;-0.58707327704333189810625981408520601689815521240234375]
      mask Display: e = 0.06;c1 = [120 150 230]/255;c2 = ([120 150 230]+0)/383;c3 = ([120 150 230]+128)/383;patch([0 1 1 0],[0 0 1 1],c1);patch([0 1 1 1-e 1-e 0+e],[0 0 1 1-e 0+e 0+e],c2);patch([0 0 1 1-e 0+e 0+e],[0 1 1 1-e 1-e 0+e],c3);plot([0 1 1 0 0],[0 0 1 1 0]);disp('weights');
  "IW{2,1}(19,:)'" : Constant  Value=[0.07046361363051829862502728474282776005566120147705078125;-0.194237147921904662606351621434441767632961273193359375;-0.05859854459964385087200611224034219048917293548583984375;0.188189009886802427473639909294433891773223876953125;0.207312890856662657146358696991228498518466949462890625;-0.16010608735028231119912334179389290511608123779296875;-0.323450370266667841523400284131639637053012847900390625;0.319792487955950999189980166192981414496898651123046875;0.77020976601191570853899293069844134151935577392578125;0.405372722881808644768142357861506752669811248779296875;-0.453619426184289020742568254718207754194736480712890625;0.57316903390399265294519182134536094963550567626953125;-0.63652072471207976622764590501901693642139434814453125;-0.59669595570767064440786953127826564013957977294921875;0.11680621200215608734840344595795613713562488555908203125;-0.61660827810789020642090463297790847718715667724609375;0.582426174097647741945138477603904902935028076171875;-0.592587906919103790670533271622844040393829345703125;0.25811811199750367418204177738516591489315032958984375;0.248210958819145732778821411557146348059177398681640625]
      mask Display: e = 0.06;c1 = [120 150 230]/255;c2 = ([120 150 230]+0)/383;c3 = ([120 150 230]+128)/383;patch([0 1 1 0],[0 0 1 1],c1);patch([0 1 1 1-e 1-e 0+e],[0 0 1 1-e 0+e 0+e],c2);patch([0 0 1 1-e 0+e 0+e],[0 1 1 1-e 1-e 0+e],c3);plot([0 1 1 0 0],[0 0 1 1 0]);disp('weights');
  "IW{2,1}(2,:)'" : Constant  Value=[-0.6334682991433575605100259053870104253292083740234375;0.92678871324707545742427328150370158255100250244140625;0.0573726512717613601477495421931962482631206512451171875;-0.488694447641380147473455508588813245296478271484375;0.2231438468912123329612740008087712340056896209716796875;-0.94217035623477174421935842474340461194515228271484375;-0.07491742171325192767294964824031922034919261932373046875;-0.73774262351045560848206150694750249385833740234375;0.5297531676274960243944178728270344436168670654296875;-0.486429041246749738203192237051553092896938323974609375;0.4500989608637320227302325292839668691158294677734375;0.60298661980059387044406093991710804402828216552734375;-0.84997943441959489252468529230100102722644805908203125;0.90387846202443722365416078901034779846668243408203125;0.4492295550298284201318210762110538780689239501953125;0.272024256827873844866161334721255116164684295654296875;0.262021920088403137416577237672754563391208648681640625;-0.27118539081706583004915955825708806514739990234375;0.219586674029197126412071838785777799785137176513671875;-0.1704454619294235584447960718534886837005615234375]
      mask Display: e = 0.06;c1 = [120 150 230]/255;c2 = ([120 150 230]+0)/383;c3 = ([120 150 230]+128)/383;patch([0 1 1 0],[0 0 1 1],c1);patch([0 1 1 1-e 1-e 0+e],[0 0 1 1-e 0+e 0+e],c2);patch([0 0 1 1-e 0+e 0+e],[0 1 1 1-e 1-e 0+e],c3);plot([0 1 1 0 0],[0 0 1 1 0]);disp('weights');
  "IW{2,1}(20,:)'" : Constant  Value=[-0.9814728081012498162039037197246216237545013427734375;-0.1265510121834192702738874913848121650516986846923828125;0.8730812149692546153545436027343384921550750732421875;-0.30675256301760811528112071755458600819110870361328125;0.1876621244917760777948245731749921105802059173583984375;0.51091005870839600877530983780161477625370025634765625;0.91629257951730125331124554577399976551532745361328125;0.71136286185388153402442412698292173445224761962890625;1.0948803721118025578107335604727268218994140625;0.53238080453134550840132988014374859631061553955078125;0.182133766658239160118881727612460963428020477294921875;-0.60238941481554852952484679917688481509685516357421875;0.07416318349215476890545772903351462446153163909912109375;-0.9242067276739003300889407910290174186229705810546875;0.77783468653463117004065452420036308467388153076171875;0.56529273677596325597960458253510296344757080078125;-0.15091848475803548712548263210919685661792755126953125;0.7665099328280735591079064761288464069366455078125;-0.83336675813816263325151112439925782382488250732421875;-0.546717025350480501089123208657838404178619384765625]
      mask Display: e = 0.06;c1 = [120 150 230]/255;c2 = ([120 150 230]+0)/383;c3 = ([120 150 230]+128)/383;patch([0 1 1 0],[0 0 1 1],c1);patch([0 1 1 1-e 1-e 0+e],[0 0 1 1-e 0+e 0+e],c2);patch([0 0 1 1-e 0+e 0+e],[0 1 1 1-e 1-e 0+e],c3);plot([0 1 1 0 0],[0 0 1 1 0]);disp('weights');
  "IW{2,1}(3,:)'" : Constant  Value=[-0.1445408738557862615703442088488372974097728729248046875;0.326526681380165884061028691576211713254451751708984375;-0.95504213665282644551979274183395318686962127685546875;0.68788397326304140388941732453531585633754730224609375;-0.5773216690097811021331608571927063167095184326171875;0.160033696894065824434250089325360022485256195068359375;0.1770070661263923594841429576263180933892726898193359375;-0.315299527012067926090566061247955076396465301513671875;0.73127027360280283385662869477528147399425506591796875;-0.1284071961474138046099824350676499307155609130859375;-0.1952927482164569517042451707311556674540042877197265625;-0.11108254379797155575460010368260554969310760498046875;-0.205865628963992686184525382486754097044467926025390625;0.84557879157271553793862040038220584392547607421875;-0.041777842188174409143730514415437937714159488677978515625;-0.64570002884290766953512274994864128530025482177734375;0.67659647216451268558756737547810189425945281982421875;-0.86938582387410356933088451114599592983722686767578125;-0.47084259769850833610149720698245801031589508056640625;0.1531416133759070097308807589797652326524257659912109375]
      mask Display: e = 0.06;c1 = [120 150 230]/255;c2 = ([120 150 230]+0)/383;c3 = ([120 150 230]+128)/383;patch([0 1 1 0],[0 0 1 1],c1);patch([0 1 1 1-e 1-e 0+e],[0 0 1 1-e 0+e 0+e],c2);patch([0 0 1 1-e 0+e 0+e],[0 1 1 1-e 1-e 0+e],c3);plot([0 1 1 0 0],[0 0 1 1 0]);disp('weights');
  "IW{2,1}(4,:)'" : Constant  Value=[-0.90321120424806389248573168515576981008052825927734375;-0.44989079073882953796470474117086268961429595947265625;0.1865294136478721498395572098161210305988788604736328125;0.11480557319521011994112313914229162037372589111328125;-0.681900175852112599983456675545312464237213134765625;0.4626104593894038163881532454979605972766876220703125;-0.8383014818324523442782947313389740884304046630859375;-0.6965466424479720419782324825064279139041900634765625;0.645802533770557740666617974056862294673919677734375;-0.361640210757333047109085555348428897559642791748046875;-0.3112026327493728761197644416824914515018463134765625;-0.1819738095936847821487702958620502613484859466552734375;0.6316598868653617859791893351939506828784942626953125;0.6839199567801637069663911461248062551021575927734375;-0.570799881000260800334444866166450083255767822265625;-0.373914923993502956722778662879136390984058380126953125;0.8967940601636292807796735360170714557170867919921875;0.501682819769922350161550639313645660877227783203125;0.1525606696810857254575921615469269454479217529296875;-0.385986863817636471907235318212769925594329833984375]
      mask Display: e = 0.06;c1 = [120 150 230]/255;c2 = ([120 150 230]+0)/383;c3 = ([120 150 230]+128)/383;patch([0 1 1 0],[0 0 1 1],c1);patch([0 1 1 1-e 1-e 0+e],[0 0 1 1-e 0+e 0+e],c2);patch([0 0 1 1-e 0+e 0+e],[0 1 1 1-e 1-e 0+e],c3);plot([0 1 1 0 0],[0 0 1 1 0]);disp('weights');
  "IW{2,1}(5,:)'" : Constant  Value=[-0.166937573250084458909014983873930759727954864501953125;0.2233795993243445909826050410629250109195709228515625;0.956240460801367486709523291210643947124481201171875;0.145260764334145198173331436919397674500942230224609375;0.33880537144446332131764165751519612967967987060546875;0.3403866886276052383664136868901550769805908203125;0.0683292404698138955421171658599632792174816131591796875;0.62650891370077477215971839541452936828136444091796875;0.527456489075092349594342522323131561279296875;0.1060546501498082772041442467525484971702098846435546875;-0.71292124548859481247831126893288455903530120849609375;-0.6711295362029658928548769836197607219219207763671875;0.053355634705374237192199160517702694050967693328857421875;0.276615009132039790795687395075219683349132537841796875;0.056360665822972270955215634558044257573783397674560546875;0.48258751828141155382212446056655608117580413818359375;-0.03455926506720086166524197324179112911224365234375;-0.261369222235208364946146275542560033500194549560546875;0.10674685598365067640269643334249849431216716766357421875;-0.042621963182308729434222271947874105535447597503662109375]
      mask Display: e = 0.06;c1 = [120 150 230]/255;c2 = ([120 150 230]+0)/383;c3 = ([120 150 230]+128)/383;patch([0 1 1 0],[0 0 1 1],c1);patch([0 1 1 1-e 1-e 0+e],[0 0 1 1-e 0+e 0+e],c2);patch([0 0 1 1-e 0+e 0+e],[0 1 1 1-e 1-e 0+e],c3);plot([0 1 1 0 0],[0 0 1 1 0]);disp('weights');
  "IW{2,1}(6,:)'" : Constant  Value=[-0.944774469369274783048240351490676403045654296875;-0.62101489446495861113106684570084325969219207763671875;-0.034040015706884252377761868046945892274379730224609375;0.65658102103979010255585535560385324060916900634765625;0.361632017762921142978171928916708566248416900634765625;-0.80187875979387535085862737105344422161579132080078125;0.5398431405581642916757800776395015418529510498046875;0.220851690491756180723115221553598530590534210205078125;-0.481205490615749964522507298170239664614200592041015625;-0.393190381992500503915977105862111784517765045166015625;0.12353753038502467143100460589266731403768062591552734375;-0.8274185798351847420661897558602504432201385498046875;0.91854686651528882901374117864179424941539764404296875;0.71401946618424150248216619729646481573581695556640625;-0.86250132567641235592503790030605159699916839599609375;0.40984708670698299926016261451877653598785400390625;-0.86866121592017453423295592074282467365264892578125;0.261953486860291129278976995919947512447834014892578125;0.855047490004213983638692297972738742828369140625;-0.385314508440096015196019152426742948591709136962890625]
      mask Display: e = 0.06;c1 = [120 150 230]/255;c2 = ([120 150 230]+0)/383;c3 = ([120 150 230]+128)/383;patch([0 1 1 0],[0 0 1 1],c1);patch([0 1 1 1-e 1-e 0+e],[0 0 1 1-e 0+e 0+e],c2);patch([0 0 1 1-e 0+e 0+e],[0 1 1 1-e 1-e 0+e],c3);plot([0 1 1 0 0],[0 0 1 1 0]);disp('weights');
  "IW{2,1}(7,:)'" : Constant  Value=[-0.91167275196492714162133097488549537956714630126953125;0.1649973582055494769615933137174579314887523651123046875;-0.328431977699657651204034891634364612400531768798828125;0.51845694174093981398954156247782520949840545654296875;-0.305976022369276845491725680403760634362697601318359375;-0.631785528193497203375272874836809933185577392578125;-0.677002078264953954800375868217088282108306884765625;0.263863923762659602356706045611645095050334930419921875;0.835506794267476760040835870313458144664764404296875;0.6740078225658667765429754581418819725513458251953125;-0.62097122366872692378336751062306575477123260498046875;0.6082491200454980262435356053174473345279693603515625;-0.313050454405888689546344494374352507293224334716796875;0.56519883127811298972886788760661147534847259521484375;-0.1236515153985850712370364590242388658225536346435546875;0.335802237325357022523775185618433170020580291748046875;0.078188977804448278607907241166685707867145538330078125;0.566740194000250330219614625093527138233184814453125;0.382370217057389660819666232782765291631221771240234375;0.75745378788854555995868622630950994789600372314453125]
      mask Display: e = 0.06;c1 = [120 150 230]/255;c2 = ([120 150 230]+0)/383;c3 = ([120 150 230]+128)/383;patch([0 1 1 0],[0 0 1 1],c1);patch([0 1 1 1-e 1-e 0+e],[0 0 1 1-e 0+e 0+e],c2);patch([0 0 1 1-e 0+e 0+e],[0 1 1 1-e 1-e 0+e],c3);plot([0 1 1 0 0],[0 0 1 1 0]);disp('weights');
  "IW{2,1}(8,:)'" : Constant  Value=[-0.713611853334687129546409778413362801074981689453125;0.52121236155290595615241500127012841403484344482421875;0.491300192410358105288281649336568079888820648193359375;-0.1462475279709091469104720317773171700537204742431640625;-0.91188347367732613957258536174776963889598846435546875;0.425200090697220256519273107187473215162754058837890625;0.30261069970335319201382162646041251718997955322265625;0.4267733277685399340128924450254999101161956787109375;0.41932358196298713526317669675336219370365142822265625;0.2081223136451248734157815079015563242137432098388671875;-0.92474049533427804536955818548449315130710601806640625;0.4884477163367222374290577135980129241943359375;0.183462226348819201771078724050312303006649017333984375;0.643218719024775342774091768660582602024078369140625;-0.15376803412565032136427589648519642651081085205078125;0.70471760382090298246993143038707785308361053466796875;-0.498912658707008349612266329131671227514743804931640625;0.343824965148131378445128802923136390745639801025390625;0.70978541974004538683828968714806251227855682373046875;0.1595755352996443832136463925053249113261699676513671875]
      mask Display: e = 0.06;c1 = [120 150 230]/255;c2 = ([120 150 230]+0)/383;c3 = ([120 150 230]+128)/383;patch([0 1 1 0],[0 0 1 1],c1);patch([0 1 1 1-e 1-e 0+e],[0 0 1 1-e 0+e 0+e],c2);patch([0 0 1 1-e 0+e 0+e],[0 1 1 1-e 1-e 0+e],c3);plot([0 1 1 0 0],[0 0 1 1 0]);disp('weights');
  "IW{2,1}(9,:)'" : Constant  Value=[-0.562809047254745120625329946051351726055145263671875;-0.357046779677132108954396016997634433209896087646484375;-0.8334839334025285761953227847698144614696502685546875;-0.7473888012409160008786557227722369134426116943359375;-0.17920576454376135888679755225894041359424591064453125;0.028579765540793992950607815828334423713386058807373046875;0.6443725540377760463428558068699203431606292724609375;0.1366449239331770926231257590188761241734027862548828125;0.62182942014198483438036646475666202604770660400390625;0.709658313848482880104029391077347099781036376953125;0.54926611867172014935789547962485812604427337646484375;0.00974681605083274442413721061484466190449893474578857421875;-0.6195418076801504358996908194967545568943023681640625;-0.80446999672437347062015078336116857826709747314453125;-0.61039855307224322178427655671839602291584014892578125;-0.446666574136407479311827728452044539153575897216796875;-0.449969585590900111871093258741893805563449859619140625;-0.05023121576061283233283205618135980330407619476318359375;-0.91348636431332064233856726787053048610687255859375;-0.396683439384820812900755981900147162377834320068359375]
      mask Display: e = 0.06;c1 = [120 150 230]/255;c2 = ([120 150 230]+0)/383;c3 = ([120 150 230]+128)/383;patch([0 1 1 0],[0 0 1 1],c1);patch([0 1 1 1-e 1-e 0+e],[0 0 1 1-e 0+e 0+e],c2);patch([0 0 1 1-e 0+e 0+e],[0 1 1 1-e 1-e 0+e],c3);plot([0 1 1 0 0],[0 0 1 1 0]);disp('weights');
  Mux : Mux  Inputs=20
      mask Display: e = 0.06;c1 = [120 150 230]/255;c2 = ([120 150 230]+0)/383;c3 = ([120 150 230]+128)/383;patch([0 1 1 0],[0 0 1 1],c1);patch([0 1 1 1-e 1-e 0+e],[0 0 1 1-e 0+e 0+e],c2);patch([0 0 1 1-e 0+e 0+e],[0 1 1 1-e 1-e 0+e],c3);plot([0 1 1 0 0],[0 0 1 1 0]);disp('Mux');
  dotprod{1..20} (20 alike) : neural/Weight Functions/dotprod
  "lz{2,1}" : Outport
      mask Display: e = 0.06;c1 = [120 230 180]/255;c2 = ([120 230 180]+0)/(256+128);c3 = ([120 230 180]+128)/(256+128);patch([0 1 1 0],[0 0 1 1],c1);patch([0 1 1 1-e 1-e 0+e],[0 0 1 1-e 0+e 0+e],c2);patch([0 0 1 1-e 0+e 0+e],[0 1 1 1-e 1-e 0+e],c3);plot([0 1 1 0 0],[0 0 1 1 0]);
  wires:
  Mux/1 -> "lz{2,1}"/1
  dotprod20/1 -> Mux/20
  "IW{2,1}(20,:)'"/1 -> dotprod20/1
  dotprod19/1 -> Mux/19
  "IW{2,1}(19,:)'"/1 -> dotprod19/1
  dotprod18/1 -> Mux/18
  "IW{2,1}(18,:)'"/1 -> dotprod18/1
  dotprod17/1 -> Mux/17
  "IW{2,1}(17,:)'"/1 -> dotprod17/1
  dotprod16/1 -> Mux/16
  "IW{2,1}(16,:)'"/1 -> dotprod16/1
  dotprod15/1 -> Mux/15
  "IW{2,1}(15,:)'"/1 -> dotprod15/1
  dotprod14/1 -> Mux/14
  "IW{2,1}(14,:)'"/1 -> dotprod14/1
  dotprod13/1 -> Mux/13
  "IW{2,1}(13,:)'"/1 -> dotprod13/1
  dotprod12/1 -> Mux/12
  "IW{2,1}(12,:)'"/1 -> dotprod12/1
  dotprod11/1 -> Mux/11
  "IW{2,1}(11,:)'"/1 -> dotprod11/1
  dotprod10/1 -> Mux/10
  "IW{2,1}(10,:)'"/1 -> dotprod10/1
  dotprod9/1 -> Mux/9
  "IW{2,1}(9,:)'"/1 -> dotprod9/1
  dotprod8/1 -> Mux/8
  "IW{2,1}(8,:)'"/1 -> dotprod8/1
  dotprod7/1 -> Mux/7
  "IW{2,1}(7,:)'"/1 -> dotprod7/1
  dotprod6/1 -> Mux/6
  "IW{2,1}(6,:)'"/1 -> dotprod6/1
  dotprod5/1 -> Mux/5
  "IW{2,1}(5,:)'"/1 -> dotprod5/1
  dotprod4/1 -> Mux/4
  "IW{2,1}(4,:)'"/1 -> dotprod4/1
  dotprod3/1 -> Mux/3
  "IW{2,1}(3,:)'"/1 -> dotprod3/1
  dotprod2/1 -> Mux/2
  "IW{2,1}(2,:)'"/1 -> dotprod2/1
  dotprod1/1 -> Mux/1
  "ad{2,1}"/1 -> dotprod20/2, dotprod19/2, dotprod18/2, dotprod17/2, dotprod16/2, dotprod15/2, dotprod14/2, dotprod13/2, dotprod12/2, dotprod11/2, dotprod10/2, dotprod9/2, dotprod8/2, dotprod7/2, dotprod6/2, dotprod5/2, dotprod4/2, dotprod3/2, dotprod2/2, dotprod1/2
  "IW{2,1}(1,:)'"/1 -> dotprod1/1

== system ClosedLoop_ACCsim/Controller 7x20/Layer 3/Delays 1 ==
  "p{3}" : Inport  PortDimensions=20
      mask Display: e = 0.06;c1 = [120 230 180]/255;c2 = ([120 230 180]+0)/(256+128);c3 = ([120 230 180]+128)/(256+128);patch([0 1 1 0],[0 0 1 1],c1);patch([0 1 1 1-e 1-e 0+e],[0 0 1 1-e 0+e 0+e],c2);patch([0 0 1 1-e 0+e 0+e],[0 1 1 1-e 1-e 0+e],c3);plot([0 1 1 0 0],[0 0 1 1 0]);
  mux : Mux  Inputs=1
      mask Display: e = 0.06;c1 = [120 150 230]/255;c2 = ([120 150 230]+0)/383;c3 = ([120 150 230]+128)/383;patch([0 1 1 0],[0 0 1 1],c1);patch([0 1 1 1-e 1-e 0+e],[0 0 1 1-e 0+e 0+e],c2);patch([0 0 1 1-e 0+e 0+e],[0 1 1 1-e 1-e 0+e],c3);plot([0 1 1 0 0],[0 0 1 1 0]);disp('Mux')
  "pd{3,2}" : Outport
      mask Display: e = 0.06;c1 = [120 230 180]/255;c2 = ([120 230 180]+0)/(256+128);c3 = ([120 230 180]+128)/(256+128);patch([0 1 1 0],[0 0 1 1],c1);patch([0 1 1 1-e 1-e 0+e],[0 0 1 1-e 0+e 0+e],c2);patch([0 0 1 1-e 0+e 0+e],[0 1 1 1-e 1-e 0+e],c3);plot([0 1 1 0 0],[0 0 1 1 0]);
  wires:
  mux/1 -> "pd{3,2}"/1
  "p{3}"/1 -> mux/1
